simulink model "SImulink_final_test"  (R2022b)
settings: Solver=FixedStepAuto  StartTime=0.0  StopTime=10  FixedStep=1/30  RelTol=1e-3
undefined symbols (not defined in the file or in its folder): Rec, SDTV, Y, Z
libraries: robotlib x4, nvidiaAVlib x2, visionconversions x2, visionanalysis x2
settings Model: Creator=Daven  LastModifiedBy=Daven

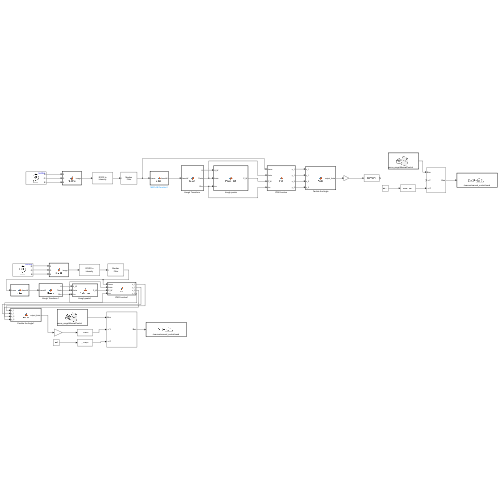
[thumbnail: Simulink's stored preview of the top-level diagram]
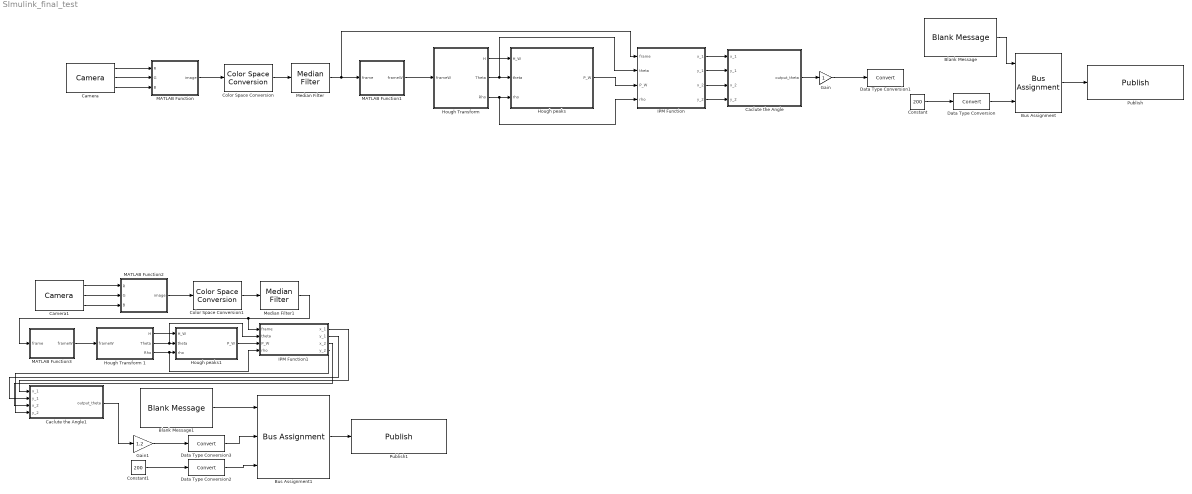
== system SImulink_final_test ==
  Blank Message : robotlib/Blank Message  messageClass=Message  entityType=mavros_msgs/ManualControl  messageType=mavros_msgs/ManualControl  SampleTime=0.02  legacyBusStruct=off
      settings: LibrarySourceBlock=roslib/ROS/Blank Message
  Blank Message1 : robotlib/Blank Message  messageClass=Message  entityType=mavros_msgs/ManualControl  messageType=mavros_msgs/ManualControl  SampleTime=0.02  legacyBusStruct=off
      settings: LibrarySourceBlock=roslib/ROS/Blank Message
  Bus Assignment : BusAssignment  AssignedSignals=Y,Z
  Bus Assignment1 : BusAssignment  AssignedSignals=Y,Z
  Caclute the Angle : MATLAB Function  TreatAsAtomicUnit=on
  Caclute the Angle1 : MATLAB Function  TreatAsAtomicUnit=on
  Camera : nvidiaAVlib/Camera  CameraName=C270 HD WEBCAM  ImageSize=[ 320, 240 ]  SampleTime=1/30  SimulateUsing=Code generation
  Camera1 : nvidiaAVlib/Camera  CameraName=C270 HD WEBCAM  ImageSize=[ 320, 240 ]  SampleTime=1/30  SimulateUsing=Code generation
  Color Space Conversion : visionconversions/Color Space  Conversion  conversion=Obsolete  conversionActive=R'G'B' to intensity  wp_str=D65  rec=Rec. 601 (SDTV)  sys=1125/60/2:1  imagePorts=One multidimensional signal
  Color Space Conversion1 : visionconversions/Color Space  Conversion  conversion=Obsolete  conversionActive=R'G'B' to intensity  wp_str=D65  rec=Rec. 601 (SDTV)  sys=1125/60/2:1  imagePorts=One multidimensional signal
  Constant : Constant  Value=200  SampleTime=0.02
  Constant1 : Constant  Value=200  SampleTime=0.02
  Data Type Conversion{,1..3} (4 alike) : DataTypeConversion  SaturateOnIntegerOverflow=off  RndMeth=Floor
  Gain : Gain
  Gain1 : Gain  Gain=1.2
  "Hough Transform " : MATLAB Function  TreatAsAtomicUnit=on
  Hough Transform 1 : MATLAB Function  TreatAsAtomicUnit=on
  Hough peaks : MATLAB Function  TreatAsAtomicUnit=on
  Hough peaks1 : MATLAB Function  TreatAsAtomicUnit=on
  IPM Function : MATLAB Function  TreatAsAtomicUnit=on
  IPM Function1 : MATLAB Function  TreatAsAtomicUnit=on
  MATLAB Function : MATLAB Function  TreatAsAtomicUnit=on
  MATLAB Function1 : MATLAB Function  TreatAsAtomicUnit=on
  MATLAB Function2 : MATLAB Function  TreatAsAtomicUnit=on
  MATLAB Function3 : MATLAB Function  TreatAsAtomicUnit=on
  Median Filter : visionanalysis/Median Filter  nghbood=[10 10 ]  outSize=Same as input port I  padType=Constant  padSrc=Specify via dialog  padVal=0  roundingMode=Floor  overflowMode=off
  Median Filter1 : visionanalysis/Median Filter  nghbood=[10 10 ]  outSize=Same as input port I  padType=Constant  padSrc=Specify via dialog  padVal=0  roundingMode=Floor  overflowMode=off
  Publish : robotlib/Publish  topicSource=Select from ROS network  topic=/mavros/manual_control/send  messageType=mavros_msgs/ManualControl  legacyBusStruct=off  messageQueueLength=1
      settings: LibrarySourceBlock=roslib/ROS/Publish
  Publish1 : robotlib/Publish  topicSource=Select from ROS network  topic=/mavros/manual_control/send  messageType=mavros_msgs/ManualControl  legacyBusStruct=off  messageQueueLength=1
      settings: LibrarySourceBlock=roslib/ROS/Publish
  wires:
  Camera/1 -> MATLAB Function/1(R)
  Camera/2 -> MATLAB Function/2(G)
  Camera/3 -> MATLAB Function/3(B)
  MATLAB Function/1(image) -> Color Space Conversion/1
  Color Space Conversion/1 -> Median Filter/1
  Median Filter/1 -> IPM Function/1(frame), MATLAB Function1/1(frame)
  "Hough Transform "/3(Rho) -> IPM Function/4(rho), Hough peaks/3(rho)
  "Hough Transform "/1(H) -> Hough peaks/1(H_W)
  "Hough Transform "/2(Theta) -> IPM Function/2(theta), Hough peaks/2(theta)
  Hough peaks/1(P_W) -> IPM Function/3(P_W)
  MATLAB Function1/1(frameW) -> "Hough Transform "/1(frameW)
  IPM Function/1(x_1) -> Caclute the Angle/1(x_1)
  IPM Function/2(y_1) -> Caclute the Angle/2(y_1)
  IPM Function/3(x_2) -> Caclute the Angle/3(x_2)
  IPM Function/4(y_2) -> Caclute the Angle/4(y_2)
  Caclute the Angle/1(output_theta) -> Gain/1
  Gain/1 -> Data Type Conversion1/1
  Bus Assignment/1 -> Publish/1
  Constant/1 -> Data Type Conversion/1
  Data Type Conversion/1 -> Bus Assignment/3
  Blank Message/1 -> Bus Assignment/1
  Constant1/1 -> Data Type Conversion2/1
  Blank Message1/1 -> Bus Assignment1/1
  Bus Assignment1/1 -> Publish1/1
  Gain1/1 -> Data Type Conversion3/1
  Camera1/1 -> MATLAB Function2/1(R)
  Data Type Conversion2/1 -> Bus Assignment1/3
  Camera1/3 -> MATLAB Function2/3(B)
  MATLAB Function2/1(image) -> Color Space Conversion1/1
  Color Space Conversion1/1 -> Median Filter1/1
  Camera1/2 -> MATLAB Function2/2(G)
  Median Filter1/1 -> IPM Function1/1(frame), MATLAB Function3/1(frame)
  MATLAB Function3/1(frameW) -> Hough Transform 1/1(frameW)
  Hough Transform 1/1(H) -> Hough peaks1/1(H_W)
  Hough Transform 1/2(Theta) -> IPM Function1/2(theta), Hough peaks1/2(theta)
  Hough Transform 1/3(Rho) -> IPM Function1/4(rho), Hough peaks1/3(rho)
  Hough peaks1/1(P_W) -> IPM Function1/3(P_W)
  IPM Function1/1(x_1) -> Caclute the Angle1/1(x_1)
  IPM Function1/2(y_1) -> Caclute the Angle1/2(y_1)
  IPM Function1/3(x_2) -> Caclute the Angle1/3(x_2)
  IPM Function1/4(y_2) -> Caclute the Angle1/4(y_2)
  Data Type Conversion3/1 -> Bus Assignment1/2
  Caclute the Angle1/1(output_theta) -> Gain1/1

== matlab function SImulink_final_test/IPM Function1 ==
  data: frame input; theta input; P_W input; rho input; x_1 output; y_1 output; x_2 output; y_2 output
function  [x_1,y_1,x_2,y_2]=IPM(frame,theta,P_W,rho)
lines_WL = houghlines(frame,theta,rho,P_W,'FillGap',3000,'MinLength',20);

imshow(frame); 
hold on

for k = 1:length(lines_WL)% 車道線右側線段連線
    xy = [lines_WL(k).point1; lines_WL(k).point2];
    plot(xy(:,1),xy(:,2),'LineWidth',2,'Color','green');

    % Plot beginnings and ends of lines
    plot(xy(1,1),xy(1,2),'x','LineWidth',2,'Color','yellow');
    plot(xy(2,1),xy(2,2),'x','LineWidth',2,'Color','red');
    axis on 
end

Center_x1 = (xy(1,1)+XY(2,1))/2;
Center_y1 = (xy(1,2)+XY(2,2))/2;
Center_x2 = (xy(2,1)+XY(1,1))/2;
Center_y2 = (xy(2,2)+XY(1,2))/2;
plot([Center_x1,Center_x2],[Center_y1,Center_y2],'LineWidth',2,'Color','blue');
xline(160);
hold off

n = 240/100 ; % 單位是 pixel/mm   
m = 320/100 ; % 單位是pixel/mm
l = 27.5/100 ;% 單位為公尺
d = -(1.5/100);% 單位為公尺
h = 8.5/100   ;% 單位為公尺
gamma = 0 ; % 單位為度數
theta = deg2rad(23); % 單位為弧度
a_ver = deg2rad(34); % 單位為弧度
a_hor = deg2rad(34); % 單位為弧度
u_1 = Center_y1/100;
v_1 = Center_x1/100;
u_2 = Center_y2/100;
v_2 = Center_x2/100;

x_1 = h*cot(((theta-a_ver) + ((u_1*2*a_ver)/(n-1))))*cos(((gamma-a_hor) + ((v_1*2*a_hor)/(m-1))))+l;
y_1 = h*cot(((theta-a_ver) + ((u_1*2*a_ver)/(n-1))))*sin(((gamma-a_hor) + ((v_1*2*a_hor)/(m-1))))+d;
x_2 = h*cot(((theta-a_ver) + ((u_2*2*a_ver)/(n-1))))*cos(((gamma-a_hor) + ((v_2*2*a_hor)/(m-1))))+l;
y_2 = h*cot(((theta-a_ver) + ((u_2*2*a_ver)/(n-1))))*sin(((gamma-a_hor) + ((v_2*2*a_hor)/(m-1))))+d;

== matlab function SImulink_final_test/MATLAB Function2 ==
  data: R input; image output; G input; B input
function image  = rgb2Img(R,G,B)
image = coder.nullcopy(uint8(zeros(size(R,1),size(R,2),3)));
image(:,:,1) = R;
image(:,:,2) = G;
image(:,:,3) = B;
end

== matlab function SImulink_final_test/MATLAB Function3 ==
  data: frame input; frameW output
function frameW  = edge( frame)

frameW = edge(frame,'canny',0.3)
frameW = bwareaopen(frameW,15)

== matlab function SImulink_final_test/MATLAB Function1 ==
  data: frame input; frameW output
function frameW  = edge( frame)

frameW = edge(frame,'canny',0.3)
frameW = bwareaopen(frameW,15)

== matlab function SImulink_final_test/MATLAB Function ==
  data: R input; image output; G input; B input
function image  = rgb2Img(R,G,B)
image = coder.nullcopy(uint8(zeros(size(R,1),size(R,2),3)));
image(:,:,1) = R;
image(:,:,2) = G;
image(:,:,3) = B;
end

== matlab function SImulink_final_test/Caclute the Angle ==
  data: x_1 input; output_theta output; y_1 input; x_2 input; y_2 input
function output_theta = Angle(x_1,y_1,x_2,y_2)

tan_theta = (y_1-y_2)/(x_1-x_2);

angle = atan(tan_theta);
rotate_angle = angle*(180/pi);  %change to degree

if rotate_angle  < 0
    output_theta = 400+(25/2)*rotate_angle;
elseif rotate_angle > 0 
    output_theta = -400-(25/2)*rotate_angle;
else 
    output_theta = 200;
end

== matlab function SImulink_final_test/Hough Transform  ==
  data: frameW input; H output; Theta output; Rho output
function [H,Theta,Rho] = Hough(frameW)

[H,Theta,Rho]= hough(frameW)

== matlab function SImulink_final_test/Hough peaks ==
  data: H_W input; theta input; rho input; P_W output size=[480 720]
function P_W  = Peaks_plot(H_W,theta,rho)

P_W = houghpeaks(H_W,2,'threshold',2);


%----------Plotting Hough Transform and detecting Hough Peaks----------

figure('Name','Hough Peaks for White Line')
imshow(imadjust(rescale(H_W)),[],'XData',theta,'YData',rho,'InitialMagnification','fit');
xlabel('\theta (degrees)')
ylabel('\rho')
axis on
axis normal
hold on
colormap(gca,hot)

x = theta(P_W(:,2));
y = rho(P_W(:,1));
plot(x,y,'s','color','blue');
hold off

== matlab function SImulink_final_test/IPM Function ==
  data: frame input; theta input; P_W input; rho input; x_1 output; y_1 output; x_2 output; y_2 output
function  [x_1,y_1,x_2,y_2]=IPM(frame,theta,P_W,rho)
lines_WL = houghlines(frame,theta,rho,P_W,'FillGap',3000,'MinLength',20);

imshow(frame); 
hold on

for k = 1:length(lines_WL)% 車道線右側線段連線
    xy = [lines_WL(k).point1; lines_WL(k).point2];
    plot(xy(:,1),xy(:,2),'LineWidth',2,'Color','green');

    % Plot beginnings and ends of lines
    plot(xy(1,1),xy(1,2),'x','LineWidth',2,'Color','yellow');
    plot(xy(2,1),xy(2,2),'x','LineWidth',2,'Color','red');
    axis on 
end

Center_x1 = (xy(1,1)+XY(2,1))/2;
Center_y1 = (xy(1,2)+XY(2,2))/2;
Center_x2 = (xy(2,1)+XY(1,1))/2;
Center_y2 = (xy(2,2)+XY(1,2))/2;
plot([Center_x1,Center_x2],[Center_y1,Center_y2],'LineWidth',2,'Color','blue');
xline(160);
hold off

n = 240/100 ; % 單位是 pixel/mm   
m = 320/100 ; % 單位是pixel/mm
l = 27.5/100 ;% 單位為公尺
d = -(1.5/100);% 單位為公尺
h = 8.5/100   ;% 單位為公尺
gamma = 0 ; % 單位為度數
theta = deg2rad(23); % 單位為弧度
a_ver = deg2rad(34); % 單位為弧度
a_hor = deg2rad(34); % 單位為弧度
u_1 = Center_y1/100;
v_1 = Center_x1/100;
u_2 = Center_y2/100;
v_2 = Center_x2/100;

x_1 = h*cot(((theta-a_ver) + ((u_1*2*a_ver)/(n-1))))*cos(((gamma-a_hor) + ((v_1*2*a_hor)/(m-1))))+l;
y_1 = h*cot(((theta-a_ver) + ((u_1*2*a_ver)/(n-1))))*sin(((gamma-a_hor) + ((v_1*2*a_hor)/(m-1))))+d;
x_2 = h*cot(((theta-a_ver) + ((u_2*2*a_ver)/(n-1))))*cos(((gamma-a_hor) + ((v_2*2*a_hor)/(m-1))))+l;
y_2 = h*cot(((theta-a_ver) + ((u_2*2*a_ver)/(n-1))))*sin(((gamma-a_hor) + ((v_2*2*a_hor)/(m-1))))+d;

== matlab function SImulink_final_test/Caclute the Angle1 ==
  data: x_1 input; output_theta output; y_1 input; x_2 input; y_2 input
function output_theta = Angle(x_1,y_1,x_2,y_2)

tan_theta = (y_1-y_2)/(x_1-x_2);

angle = atan(tan_theta);
rotate_angle = angle*(180/pi);  %change to degree

if rotate_angle  < 0
    output_theta = 400+(25/2)*rotate_angle;
elseif rotate_angle > 0 
    output_theta = -400-(25/2)*rotate_angle;
else 
    output_theta = 200;
end

== matlab function SImulink_final_test/Hough Transform 1 ==
  data: frameW input; H output; Theta output; Rho output
function [H,Theta,Rho] = Hough(frameW)

[H,Theta,Rho]= hough(frameW)

== matlab function SImulink_final_test/Hough peaks1 ==
  data: H_W input; theta input; rho input; P_W output size=[480 720]
function P_W  = Peaks_plot(H_W,theta,rho)

P_W = houghpeaks(H_W,2,'threshold',2);


%----------Plotting Hough Transform and detecting Hough Peaks----------

figure('Name','Hough Peaks for White Line')
imshow(imadjust(rescale(H_W)),[],'XData',theta,'YData',rho,'InitialMagnification','fit');
xlabel('\theta (degrees)')
ylabel('\rho')
axis on
axis normal
hold on
colormap(gca,hot)

x = theta(P_W(:,2));
y = rho(P_W(:,1));
plot(x,y,'s','color','blue');
hold off
